simulink model "BOM_Navigation"  (R2013a)
settings: Solver=ode45  StartTime=0.0  StopTime=10.0  RelTol=1e-3
settings Model: Creator=HoangMinh  LastModifiedBy=HoangMinh

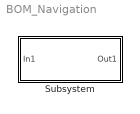
== system BOM_Navigation ==
  Subsystem : Subsystem

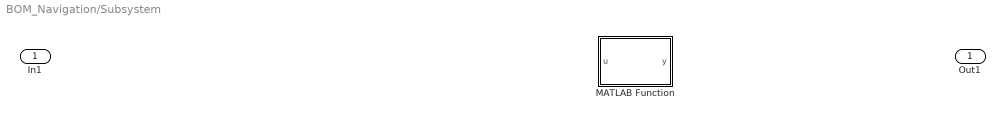
== system BOM_Navigation/Subsystem ==
  In1 : Inport
  MATLAB Function : MATLAB Function  TreatAsAtomicUnit=on
  Out1 : Outport

== matlab function BOM_Navigation/Subsystem/MATLAB Function ==
  data: u input; y output
function y = fcn(u)
%#codegen

y = u;
